simulink model "CMy_th"  (R2018b)
settings: Solver=VariableStepAuto  StartTime=0.0  StopTime=0  RelTol=1e-3
values from neighbouring files (symbols this model uses):
  alphaDeg = 5    [CMy_ts.m]
  alphas = Cmtot_2D_Tbl.Breakpoints(1).Value    [CMy_ts.m]
  betaDeg = 0    [CMy_ts.m]
  betas = 1.1*Cmtot_2D_Tbl.Breakpoints(2).Value    [CMy_ts.m]
  val = Cmtot_2D_Tbl.Table.Value    [CMy_ts.m]
settings Model: Creator=mcobb  LastModifiedBy=mcobb

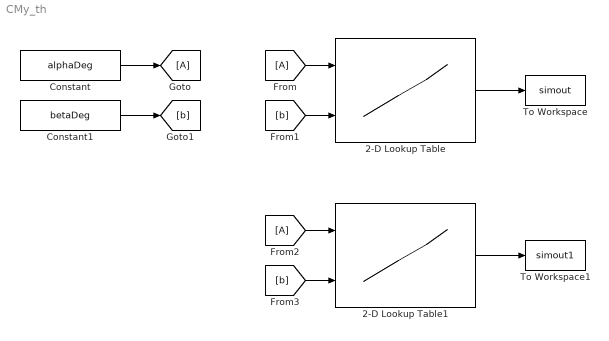
== system CMy_th ==
  2-D Lookup Table : Lookup_n-D  LookupTableObject=Cmtot_2D_Tbl  BreakpointsForDimension1=alphas  BreakpointsForDimension2=betas  Table=val  InternalRulePriority=Speed  RndMeth=Simplest  InputSameDT=on
  2-D Lookup Table1 : Lookup_n-D  DataSpecification=Lookup table object  LookupTableObject=Cmtot_2D_Tbl  BreakpointsForDimension1=alphas  BreakpointsForDimension2=betas  Table=val  InternalRulePriority=Speed  RndMeth=Simplest  InputSameDT=on
  Constant : Constant  Value=alphaDeg
  Constant1 : Constant  Value=betaDeg
  To Workspace : ToWorkspace  VariableName=simout  SaveFormat=Timeseries  SampleTime=-1
  To Workspace1 : ToWorkspace  VariableName=simout1  SaveFormat=Timeseries  SampleTime=-1
  wires:
  2-D Lookup Table/1 -> To Workspace/1
  2-D Lookup Table1/1 -> To Workspace1/1
  [A] -> 2-D Lookup Table/1
  [b] -> 2-D Lookup Table/2
  [A] -> 2-D Lookup Table1/1
  [b] -> 2-D Lookup Table1/2
  Constant/1 -> [A]
  Constant1/1 -> [b]
